simulink model "MaIA_SDCI_Temperature_Control"  (R2025b)
settings: Solver=VariableStepAuto  StartTime=0.0  StopTime=1800  RelTol=1e-3
PreLoadFcn:
  | %% MaIA_SDCI - Model Preload Callback
  | % Keep this callback intentionally minimal.
  | % All portable initialization logic lives in startup_project.m.
  | 
  | modelFile = get_param(bdroot, 'FileName');
  | 
  | if isempty(modelFile)
  |     error('MaIA_SDCI:ModelFileNotFound', ...
  |         'Unable to determine the current model file location.');
  | end
  | 
  | projectRoot = fileparts(modelFile);
  | addpath(projectRoot, '-begin');
  | rehash path;
  | startup_project(projectRoot);
InitFcn:
  | %% ============================================================
  | %  SIMULATION LAUNCH SOURCE
  | %  ============================================================
  | 
  | % false -> Run initiated directly from Simulink
  | % true  -> Run initiated from the MaIA_SDCI GUI
  | %
  | % Do not overwrite this variable if it already exists because
  | % the GUI sets it to true immediately before starting a run.
  | 
  | if ~evalin( ...
  |         'base', ...
  |         'exist(''MaIA_SDCI_RUN_FROM_GUI'',''var'')')
  | 
  |     assignin( ...
  |         'base', ...
  |         'MaIA_SDCI_RUN_FROM_GUI', ...
  |         false);
  | 
  | end
StartFcn:
  | %% MaIA_SDCI - Simulation Start Callback
  | 
  | runFromGUI = false;
  | 
  | %% Check simulation origin
  | 
  | if evalin( ...
  |         'base', ...
  |         'exist(''MaIA_SDCI_RUN_FROM_GUI'',''var'')')
  | 
  |     flagValue = evalin( ...
  |         'base', ...
  |         'MaIA_SDCI_RUN_FROM_GUI');
  | 
  |     if islogical(flagValue) || isnumeric(flagValue)
  |         runFromGUI = logical(flagValue);
  |     end
  | 
  | end
  | 
  | %% Open or focus the control application
  | 
  | launch_app;
  | 
  | %% Manual Run from Simulink
  | 
  | if ~runFromGUI
  | 
  |     drawnow;
  | 
  |     set_param( ...
  |         bdroot, ...
  |         'SimulationCommand', ...
  |         'stop');
  | 
  | end
values from neighbouring files (symbols this model uses):
  CFG = project_config()    [startup_project.m]
  ENV = environment_parameters()    [startup_project.m]
  MODEL = model_parameters()    [startup_project.m]
  SENSOR = sensor_parameters()    [startup_project.m]
libraries: fl_lib x58, nesl_utility x38, simulink x2
(part 1 of 2)
settings Model: PacingRate=100  Creator=leffe  LastModifiedBy=leffe

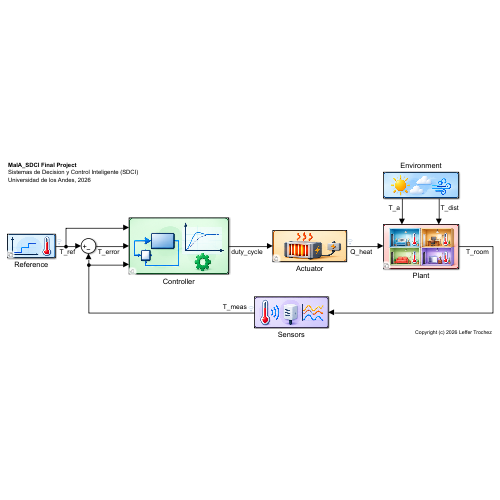
[thumbnail: Simulink's stored preview of the top-level diagram]
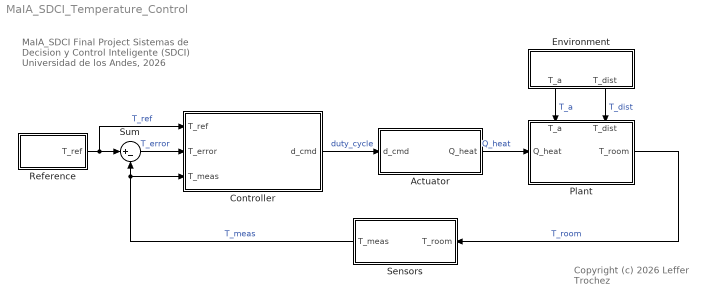
== system MaIA_SDCI_Temperature_Control ==
  note: Copyright (c) 2026 Leffer Trochez
  note: MaIA_SDCI Final Project
      | Sistemas de Decision y Control Inteligente (SDCI)
      | Universidad de los Andes, 2026
  Actuator : Subsystem  Variant=on  AllowFlexibleInterface=off
      mask Display: image('Actuador.png');
  Controller : Subsystem  Variant=on  AllowFlexibleInterface=off
      mask Display: image('Controller.png');
  Environment : Subsystem
      settings: PortSchema="{\"entries\":[{\"content\":{\"sides\":[{\"content\":{},\"type\":\"ConnectorPlacement.EquallySpacedRectSide\",\"uuid\":\"1a7bcca7-25d4-42c2-aca3-18b46478235c\"},{\"content\":{\"side\":\"RIGHT\"},\"type\":\"ConnectorPlacement.EquallySpacedRectSide\",\"uuid\":\"da09975b-28e2-4b16-92a5-057e0d52e938\"},{\"content\":{\"side\":\"TOP\"},\"type\":\"ConnectorPlacement.EquallySpacedRectSide\",\"uuid\":\"de133f6c-3388-4fad-acff-8d704dc07206\"},{\"content\":{\"connectorIds\":[\"Out1\",\"Out2\"],\"side\":\"BOTTOM\"},\"type\":\"ConnectorPlacement.EquallySpacedRectSide\",\"uuid\":\"319bfc7a-61e7-4d85-9757-ec8360a08b79\"}]},\"type\":\"ConnectorPlacement.EquallySpacedConnector\",\"uuid\":\"d277b6ce-17a2-42f7-b477-40e753a041d0\"}],\"packageUris\":[\"http://schema.mathworks.com/mf0/Connector/R2020b\"],\"version\":\"1.0\"}"
      mask Display: image('Environment.png');
  Plant : Subsystem  Variant=on  AllowFlexibleInterface=off
      settings: PortSchema="{\"entries\":[{\"content\":{\"sides\":[{\"content\":{\"connectorIds\":[\"In1\"]},\"type\":\"ConnectorPlacement.EquallySpacedRectSide\",\"uuid\":\"eba42224-8341-45a9-ac01-2acfcdf2210a\"},{\"content\":{\"connectorIds\":[\"Out1\"],\"side\":\"RIGHT\"},\"type\":\"ConnectorPlacement.EquallySpacedRectSide\",\"uuid\":\"282eb00b-7a70-45a6-85b7-dc180b696deb\"},{\"content\":{\"connectorIds\":[\"In2\",\"In3\"],\"side\":\"TOP\"},\"type\":\"ConnectorPlacement.EquallySpacedRectSide\",\"uuid\":\"41565600-1cc1-40b4-b112-8c0c6227dbf3\"}]},\"type\":\"ConnectorPlacement.EquallySpacedConnector\",\"uuid\":\"88025b6d-ed49-4509-ac82-02d3bec1907f\"}],\"packageUris\":[\"http://schema.mathworks.com/mf0/Connector/R2020b\"],\"version\":\"1.0\"}"
      mask Display: image('Plant.png');
  Reference : Subsystem  Variant=on  AllowFlexibleInterface=off
      mask Display: image('Reference.png');
  Sensors : Subsystem
      mask Display: image('Sensor.png');
  Sum : Sum  Inputs=|+-
  wires:
  Reference/1(T_ref) -> Sum/1, Controller/1(T_ref)  "T_ref"
  Sum/1 -> Controller/2(T_error)  "T_error"
  Sensors/1(T_meas) -> Controller/3(T_meas), Sum/2  "T_meas"
  Controller/1(d_cmd) -> Actuator/1(d_cmd)  "duty_cycle"
  Actuator/1(Q_heat) -> Plant/1(Q_heat)  "Q_heat"
  Plant/1(T_room) -> Sensors/1(T_room)  "T_room"
  Environment/1(T_a) -> Plant/2(T_a)  "T_a"
  Environment/2(T_dist) -> Plant/3(T_dist)  "T_dist"

== system MaIA_SDCI_Temperature_Control/Actuator ==
  d_cmd : Inport
  Block_Based : Subsystem  VariantControl=MODEL_TYPE_ID == 1
  Physics_Based : Subsystem  VariantControl=MODEL_TYPE_ID == 2
  Q_heat : Outport

== system MaIA_SDCI_Temperature_Control/Controller ==
  T_ref : Inport
  T_error : Inport  Port=2
  T_meas : Inport  Port=3
  Extremum_Seeking_Control : Subsystem  VariantControl=CONTROLLER_ID == 4
  Fuzzy_Logic : Subsystem  VariantControl=CONTROLLER_ID == 2
  Model_Predictive_Control : Subsystem  VariantControl=CONTROLLER_ID == 3
  ON_OFF : Subsystem  VariantControl=CONTROLLER_ID == 1
  Replicator_Dynamics : Subsystem  VariantControl=CONTROLLER_ID == 5
  d_cmd : Outport

== system MaIA_SDCI_Temperature_Control/Environment ==
  Ambient Temperature : Constant  Value=ENV.T_a
  Disturbance End : Step  Time=60 * ENV.disturbance.endTime  After=-ENV.disturbance.enabled * ENV.disturbance.amplitude  SampleTime=0
  Disturbance Start : Step  Time=60 * ENV.disturbance.startTime  After=ENV.disturbance.enabled * ENV.disturbance.amplitude  SampleTime=0
  Room Selection : Gain  Gain=ENV.disturbance.roomMask  Multiplication=Matrix(K*u)
  Temperature Disturbance : Sum  Inputs=|++
  T_a : Outport
  T_dist : Outport  Port=2
  tag scope: T_a=global
  wires:
  Ambient Temperature/1 -> [T_a], T_a/1
  Disturbance Start/1 -> Temperature Disturbance/1
  Disturbance End/1 -> Temperature Disturbance/2
  Temperature Disturbance/1 -> Room Selection/1
  Room Selection/1 -> T_dist/1

== system MaIA_SDCI_Temperature_Control/Plant ==
  Q_heat : Inport
  T_a : Inport  Port=2
  T_dist : Inport  Port=3
  Block_Based : Subsystem  VariantControl=MODEL_TYPE_ID == 1
  Physics_Based : Subsystem  VariantControl=MODEL_TYPE_ID == 2
  T_room : Outport

== system MaIA_SDCI_Temperature_Control/Reference ==
  Reference_1Room : Subsystem  VariantControl=CONTROLLER_ID == 4
  Reference_4Rooms : Subsystem  VariantControl=CONTROLLER_ID ~= 4
  T_ref : Outport

== system MaIA_SDCI_Temperature_Control/Sensors ==
  T_room : Inport
  Active Sensor Mask : Product
  Demux : Demux
  Mux : Mux
  Sensor Mask : Constant  Value=[1; CONTROLLER_ID ~= 4; CONTROLLER_ID ~= 4; CONTROLLER_ID ~= 4]
  Temperature Sensor 1 : Subsystem
  Temperature Sensor 2 : Subsystem
  Temperature Sensor 3 : Subsystem
  Temperature Sensor 4 : Subsystem
  T_meas : Outport
  wires:
  T_room/1 -> Demux/1
  Temperature Sensor 1/1(T_meas_1) -> Mux/1
  Demux/1 -> Temperature Sensor 1/1(T_1)
  Mux/1 -> Active Sensor Mask/1
  Sensor Mask/1 -> Active Sensor Mask/2
  Active Sensor Mask/1 -> T_meas/1
  Demux/2 -> Temperature Sensor 2/1(T_2)
  Demux/3 -> Temperature Sensor 3/1(T_3)
  Demux/4 -> Temperature Sensor 4/1(T_4)
  Temperature Sensor 2/1(T_meas_2) -> Mux/2
  Temperature Sensor 3/1(T_meas_3) -> Mux/3
  Temperature Sensor 4/1(T_meas_4) -> Mux/4

== system MaIA_SDCI_Temperature_Control/Actuator/Block_Based ==
  d_cmd : Inport
  Constant : Constant
  Constant1 : Constant  Value=0
  Demux : Demux
  Heater_1 : Subsystem
  Heater_2 : Subsystem
  Heater_3 : Subsystem
  Heater_4 : Subsystem
  Mux : Mux
  "Saturation Dynamic " : simulink/Discontinuities/Saturation Dynamic  OutMin=[]  OutMax=[]  OutDataTypeStr=Inherit: Same as second input  OutDataType=fixdt(1, 16)  OutScaling=2^-10  DoSatur=off
  Q_heat : Outport
  wires:
  Mux/1 -> Q_heat/1  "[W]"
  "Saturation Dynamic "/1 -> Demux/1  "[-]"
  d_cmd/1 -> "Saturation Dynamic "/2
  Demux/1 -> Heater_1/1(d_1)
  Heater_1/1(Q_1) -> Mux/1
  Constant/1 -> "Saturation Dynamic "/1
  Constant1/1 -> "Saturation Dynamic "/3
  Demux/2 -> Heater_2/1(d_2)
  Demux/3 -> Heater_3/1(d_3)
  Demux/4 -> Heater_4/1(d_4)
  Heater_2/1(Q_2) -> Mux/2
  Heater_3/1(Q_3) -> Mux/3
  Heater_4/1(Q_4) -> Mux/4

== system MaIA_SDCI_Temperature_Control/Actuator/Physics_Based ==
  d_cmd : Inport
  Demux : Demux
  "Duty Cycle Saturation " : simulink/Discontinuities/Saturation Dynamic  OutMin=[]  OutMax=[]  OutDataTypeStr=Inherit: Same as second input  OutDataType=fixdt(1, 16)  OutScaling=2^-10  DoSatur=off
  Heater_1 : Subsystem
  Heater_2 : Subsystem
  Heater_3 : Subsystem
  Heater_4 : Subsystem
  Lower Duty Limit : Constant  Value=0
  Mux : Mux
  Upper Duty Limit : Constant
  Q_heat : Outport
  wires:
  d_cmd/1 -> "Duty Cycle Saturation "/2
  Lower Duty Limit/1 -> "Duty Cycle Saturation "/3
  Heater_1/1(Q_1) -> Mux/1
  Upper Duty Limit/1 -> "Duty Cycle Saturation "/1
  Mux/1 -> Q_heat/1  "[W]"
  Demux/1 -> Heater_1/1(d_1)
  "Duty Cycle Saturation "/1 -> Demux/1  "[-]"
  Demux/2 -> Heater_2/1(d_2)
  Demux/3 -> Heater_3/1(d_3)
  Demux/4 -> Heater_4/1(d_4)
  Heater_2/1(Q_2) -> Mux/2
  Heater_3/1(Q_3) -> Mux/3
  Heater_4/1(Q_4) -> Mux/4

== system MaIA_SDCI_Temperature_Control/Controller/Extremum_Seeking_Control ==
  T_ref : Inport
  T_error : Inport  Port=2
  T_meas : Inport  Port=3
  d_cmd : Outport

== system MaIA_SDCI_Temperature_Control/Controller/Fuzzy_Logic ==
  T_ref : Inport
  T_error : Inport  Port=2
  T_meas : Inport  Port=3
  d_cmd : Outport

== system MaIA_SDCI_Temperature_Control/Controller/Model_Predictive_Control ==
  T_ref : Inport
  T_error : Inport  Port=2
  T_meas : Inport  Port=3
  d_cmd : Outport

== system MaIA_SDCI_Temperature_Control/Controller/ON_OFF ==
  T_ref : Inport
  T_error : Inport  Port=2
  T_meas : Inport  Port=3
  d_cmd : Outport

== system MaIA_SDCI_Temperature_Control/Controller/Replicator_Dynamics ==
  T_ref : Inport
  T_error : Inport  Port=2
  T_meas : Inport  Port=3
  d_cmd : Outport

== system MaIA_SDCI_Temperature_Control/Plant/Block_Based ==
  Q_heat : Inport
  T_a : Inport  Port=2
  T_dist : Inport  Port=3
  Building Configuration : Subsystem  Variant=on  AllowFlexibleInterface=off
  T_room : Outport
  wires:
  Building Configuration/1(T_room) -> T_room/1
  Q_heat/1 -> Building Configuration/1(Q_heat)
  T_a/1 -> Building Configuration/2(T_a)
  T_dist/1 -> Building Configuration/3(T_dist)

== system MaIA_SDCI_Temperature_Control/Plant/Physics_Based ==
  Q_heat : Inport
  T_a : Inport  Port=2
  T_dist : Inport  Port=3
  Building Configuration : Subsystem  Variant=on  AllowFlexibleInterface=off
  T_room : Outport
  wires:
  Q_heat/1 -> Building Configuration/1(Q_heat)
  T_a/1 -> Building Configuration/2(T_a)
  T_dist/1 -> Building Configuration/3(T_dist)
  Building Configuration/1(T_room) -> T_room/1

== system MaIA_SDCI_Temperature_Control/Reference/Reference_1Room ==
  Constant : Constant  Value=[CFG.reference.singleRoom; 0; 0; 0]
  T_ref : Outport
  wires:
  Constant/1 -> T_ref/1

== system MaIA_SDCI_Temperature_Control/Reference/Reference_4Rooms ==
  Constant : Constant  Value=CFG.reference.fourRooms
  T_ref : Outport
  wires:
  Constant/1 -> T_ref/1

== system MaIA_SDCI_Temperature_Control/Sensors/Temperature Sensor 1 ==
  T_1 : Inport
  Measured Temperature : Sum  Inputs=|+++
  Measurement Noise : RandomNumber  Variance=SENSOR.noiseStd(1)^2  Seed=SENSOR.seed(1)  SampleTime=SENSOR.sampleTime
  Sampling : ZeroOrderHold  SampleTime=SENSOR.sampleTime
  Sensor Dynamics Gain : Gain  Gain=1/SENSOR.tau
  Sensor Temperature : Integrator  InitialCondition=SENSOR.initialTemperature(1)
  Sensor Bias : Constant  Value=SENSOR.bias(1)
  Sum : Sum  Inputs=|+-
  T_meas_1 : Outport
  wires:
  T_1/1 -> Sum/1
  Sensor Temperature/1 -> Sum/2, Sampling/1
  Sampling/1 -> Measured Temperature/2
  Sensor Bias/1 -> Measured Temperature/3
  Measurement Noise/1 -> Measured Temperature/1
  Measured Temperature/1 -> T_meas_1/1
  Sum/1 -> Sensor Dynamics Gain/1
  Sensor Dynamics Gain/1 -> Sensor Temperature/1

== system MaIA_SDCI_Temperature_Control/Sensors/Temperature Sensor 2 ==
  T_2 : Inport
  Measured Temperature : Sum  Inputs=|+++
  Measurement Noise : RandomNumber  Variance=SENSOR.noiseStd(2)^2  Seed=SENSOR.seed(2)  SampleTime=SENSOR.sampleTime
  Sampling : ZeroOrderHold  SampleTime=SENSOR.sampleTime
  Sensor Dynamics Gain : Gain  Gain=1/SENSOR.tau
  Sensor Temperature : Integrator  InitialCondition=SENSOR.initialTemperature(2)
  Sensor Bias : Constant  Value=SENSOR.bias(2)
  Sum : Sum  Inputs=|+-
  T_meas_2 : Outport
  wires:
  T_2/1 -> Sum/1
  Sum/1 -> Sensor Dynamics Gain/1
  Measured Temperature/1 -> T_meas_2/1
  Measurement Noise/1 -> Measured Temperature/1
  Sampling/1 -> Measured Temperature/2
  Sensor Temperature/1 -> Sum/2, Sampling/1
  Sensor Bias/1 -> Measured Temperature/3
  Sensor Dynamics Gain/1 -> Sensor Temperature/1

== system MaIA_SDCI_Temperature_Control/Sensors/Temperature Sensor 3 ==
  T_3 : Inport
  Measured Temperature : Sum  Inputs=|+++
  Measurement Noise : RandomNumber  Variance=SENSOR.noiseStd(3)^2  Seed=SENSOR.seed(3)  SampleTime=SENSOR.sampleTime
  Sampling : ZeroOrderHold  SampleTime=SENSOR.sampleTime
  Sensor Dynamics Gain : Gain  Gain=1/SENSOR.tau
  Sensor Temperature : Integrator  InitialCondition=SENSOR.initialTemperature(3)
  Sensor Bias : Constant  Value=SENSOR.bias(3)
  Sum : Sum  Inputs=|+-
  T_meas_3 : Outport
  wires:
  Sensor Dynamics Gain/1 -> Sensor Temperature/1
  Sampling/1 -> Measured Temperature/2
  Measured Temperature/1 -> T_meas_3/1
  Sum/1 -> Sensor Dynamics Gain/1
  T_3/1 -> Sum/1
  Sensor Bias/1 -> Measured Temperature/3
  Sensor Temperature/1 -> Sum/2, Sampling/1
  Measurement Noise/1 -> Measured Temperature/1

== system MaIA_SDCI_Temperature_Control/Sensors/Temperature Sensor 4 ==
  T_4 : Inport
  Measured Temperature : Sum  Inputs=|+++
  Measurement Noise : RandomNumber  Variance=SENSOR.noiseStd(4)^2  Seed=SENSOR.seed(4)  SampleTime=SENSOR.sampleTime
  Sampling : ZeroOrderHold  SampleTime=SENSOR.sampleTime
  Sensor Dynamics Gain : Gain  Gain=1/SENSOR.tau
  Sensor Temperature : Integrator  InitialCondition=SENSOR.initialTemperature(4)
  Sensor Bias : Constant  Value=SENSOR.bias(4)
  Sum : Sum  Inputs=|+-
  T_meas_4 : Outport
  wires:
  Sensor Temperature/1 -> Sum/2, Sampling/1
  Measurement Noise/1 -> Measured Temperature/1
  Sensor Bias/1 -> Measured Temperature/3
  T_4/1 -> Sum/1
  Sensor Dynamics Gain/1 -> Sensor Temperature/1
  Sum/1 -> Sensor Dynamics Gain/1
  Measured Temperature/1 -> T_meas_4/1
  Sampling/1 -> Measured Temperature/2

== system MaIA_SDCI_Temperature_Control/Actuator/Block_Based/Heater_1 ==
  d_1 : Inport
  Control Window Hold : ZeroOrderHold  SampleTime=MODEL.BLOCK_BASED.ACTUATOR.controlWindow
  Cycle Quantizer : Rounding  Operator=round
  Cycle Count to Thermal Power : Gain  Gain=|
      | MODEL.BLOCK_BASED.ACTUATOR.P_rated * MODEL.BLOCK_BASED.ACTUATOR.efficiency / ...
      |     MODEL.BLOCK_BASED.ACTUATOR.cyclesPerWindow
  Duty to Cycle Count : Gain  Gain=MODEL.BLOCK_BASED.ACTUATOR.cyclesPerWindow
  Q_1 : Outport
  wires:
  d_1/1 -> Control Window Hold/1
  Duty to Cycle Count/1 -> Cycle Quantizer/1
  Control Window Hold/1 -> Duty to Cycle Count/1
  Cycle Quantizer/1 -> Cycle Count to Thermal Power/1
  Cycle Count to Thermal Power/1 -> Q_1/1

== system MaIA_SDCI_Temperature_Control/Actuator/Block_Based/Heater_2 ==
  d_2 : Inport
  Control Window Hold : ZeroOrderHold  SampleTime=MODEL.BLOCK_BASED.ACTUATOR.controlWindow
  Cycle Quantizer : Rounding  Operator=round
  Cycle Count to Thermal Power : Gain  Gain=|
      | MODEL.BLOCK_BASED.ACTUATOR.P_rated * MODEL.BLOCK_BASED.ACTUATOR.efficiency / ...
      |     MODEL.BLOCK_BASED.ACTUATOR.cyclesPerWindow
  Duty to Cycle Count : Gain  Gain=MODEL.BLOCK_BASED.ACTUATOR.cyclesPerWindow
  Q_2 : Outport
  wires:
  Cycle Quantizer/1 -> Cycle Count to Thermal Power/1
  Control Window Hold/1 -> Duty to Cycle Count/1
  Duty to Cycle Count/1 -> Cycle Quantizer/1
  d_2/1 -> Control Window Hold/1
  Cycle Count to Thermal Power/1 -> Q_2/1

== system MaIA_SDCI_Temperature_Control/Actuator/Block_Based/Heater_3 ==
  d_3 : Inport
  Control Window Hold : ZeroOrderHold  SampleTime=MODEL.BLOCK_BASED.ACTUATOR.controlWindow
  Cycle Quantizer : Rounding  Operator=round
  Cycle Count to Thermal Power : Gain  Gain=|
      | MODEL.BLOCK_BASED.ACTUATOR.P_rated * MODEL.BLOCK_BASED.ACTUATOR.efficiency / ...
      |     MODEL.BLOCK_BASED.ACTUATOR.cyclesPerWindow
  Duty to Cycle Count : Gain  Gain=MODEL.BLOCK_BASED.ACTUATOR.cyclesPerWindow
  Q_3 : Outport
  wires:
  Cycle Quantizer/1 -> Cycle Count to Thermal Power/1
  Control Window Hold/1 -> Duty to Cycle Count/1
  Duty to Cycle Count/1 -> Cycle Quantizer/1
  d_3/1 -> Control Window Hold/1
  Cycle Count to Thermal Power/1 -> Q_3/1

== system MaIA_SDCI_Temperature_Control/Actuator/Block_Based/Heater_4 ==
  d_4 : Inport
  Control Window Hold : ZeroOrderHold  SampleTime=MODEL.BLOCK_BASED.ACTUATOR.controlWindow
  Cycle Quantizer : Rounding  Operator=round
  Cycle Count to Thermal Power : Gain  Gain=|
      | MODEL.BLOCK_BASED.ACTUATOR.P_rated * MODEL.BLOCK_BASED.ACTUATOR.efficiency / ...
      |     MODEL.BLOCK_BASED.ACTUATOR.cyclesPerWindow
  Duty to Cycle Count : Gain  Gain=MODEL.BLOCK_BASED.ACTUATOR.cyclesPerWindow
  Q_4 : Outport
  wires:
  Cycle Quantizer/1 -> Cycle Count to Thermal Power/1
  Control Window Hold/1 -> Duty to Cycle Count/1
  Duty to Cycle Count/1 -> Cycle Quantizer/1
  d_4/1 -> Control Window Hold/1
  Cycle Count to Thermal Power/1 -> Q_4/1

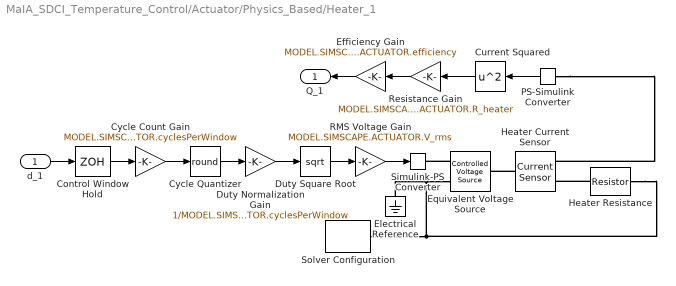
== system MaIA_SDCI_Temperature_Control/Actuator/Physics_Based/Heater_1 ==
  d_1 : Inport
  Control Window Hold : ZeroOrderHold  SampleTime=MODEL.SIMSCAPE.ACTUATOR.controlWindow
  Current Squared : Math  Operator=square
  Cycle Count Gain : Gain  Gain=MODEL.SIMSCAPE.ACTUATOR.cyclesPerWindow
  Cycle Quantizer : Rounding  Operator=round
  Duty Normalization Gain : Gain  Gain=1/MODEL.SIMSCAPE.ACTUATOR.cyclesPerWindow
  Duty Square Root : Sqrt
  Efficiency Gain : Gain  Gain=MODEL.SIMSCAPE.ACTUATOR.efficiency
  Electrical Reference : fl_lib/Electrical/Electrical Elements/Electrical Reference
  Equivalent Voltage Source : fl_lib/Electrical/Electrical Sources/Controlled Voltage Source
  Heater Resistance : fl_lib/Electrical/Electrical Elements/Resistor  R=MODEL.SIMSCAPE.ACTUATOR.R_heater Ohm  i_specify=off  i_priority=None  i=0 A  i_nominal_specify=off  i_nominal_value=1  i_nominal_unit=A  v_specify=off  v_priority=None  v=0 V  v_nominal_specify=off  v_nominal_value=1  v_nominal_unit=V
  Heater Current Sensor : fl_lib/Electrical/Electrical Sensors/Current Sensor
  PS-Simulink Converter : nesl_utility/PS-Simulink Converter  PhysicalDomain=network_engine_domain  SubClassName=ps_output  LeftPortType=input  RightPortType=output  PseudoPeriodic=off  Frequencies=[]  VectorFormat=inherit  Unit=A  AffineConversion=off
  RMS Voltage Gain : Gain  Gain=MODEL.SIMSCAPE.ACTUATOR.V_rms
  Resistance Gain : Gain  Gain=MODEL.SIMSCAPE.ACTUATOR.R_heater
  Simulink-PS Converter : nesl_utility/Simulink-PS Converter  PhysicalDomain=network_engine_domain  SubClassName=ps_input  LeftPortType=input  RightPortType=output  PseudoPeriodic=off  Frequencies=[]  NoiseDistribution=none  NoiseParameters=[]  Unit=V  AffineConversion=off  FilteringAndDerivatives=provide  SimscapeFilterOrder=1  InputFilterTimeConstant=0.001  UdotUserProvided=0
  Solver Configuration : nesl_utility/Solver Configuration  PhysicalDomain=network_engine_domain  SubClassName=solver  LeftPortType=input  RightPortType=generic  Tones=[]  Harmonics=[]  SimulateNoise=off  Profile=off  UseLocalSampling=off  EnableSwitchedLinearOptims=on  FrequencyDomain=off  UseCCode=off  RelTol=0.001  AbsTol=0.001  MinStep=1e-09  ToWorkspace=off  RevertToSquareIcSolve=off  NumHomotopyIterations=100  PhasorMode=off  PhasorModeNumHarmonics=1  ConsistencySolver=NEWTON_XTOL_AFTER_FTOL  IndexReductionMethod=DerivativeReplacement  DoDC=off  ResidualTolerance=1e-09  ConsistencyTolSource=GLOBAL  ConsistencyAbsTol=0.001  ConsistencyRelTol=0.001  ConsistencyTolFactor=0.001  UseLocalSolver=off  LocalSolverChoice=NE_BACKWARD_EULER_ADVANCER  ResolveIndetEquations=on  FunctionEvalNumThread=1  LocalSolverSampleTime=0.001  DoFixedCost=off  MaxNonlinIter=3  MaxModeIter=2  ComputeImpulses=off  ImpulseIterations=2  LinearAlgebra=auto  LinearAlgebraNumThread=0  EquationFormulation=NE_TIME_EF  DelaysMemoryBudget=1024  AutomaticFiltering=on  FilteringTimeConstant=0.001  PartitionStorageMethod=AS_NEEDED  PartitionMemoryBudget=1024  PartitionMethod=ROBUST  MultibodyUseLocalSolver=off  MultibodyLocalSolverChoice=ODE1  MultibodyLocalSolverSampleTime=0.001
  Q_1 : Outport
  wires:
  d_1/1 -> Control Window Hold/1
  Cycle Count Gain/1 -> Cycle Quantizer/1
  Control Window Hold/1 -> Cycle Count Gain/1
  Cycle Quantizer/1 -> Duty Normalization Gain/1
  Duty Normalization Gain/1 -> Duty Square Root/1
  Duty Square Root/1 -> RMS Voltage Gain/1
  RMS Voltage Gain/1 -> Simulink-PS Converter/1
  PS-Simulink Converter/1 -> Current Squared/1
  Current Squared/1 -> Resistance Gain/1
  Resistance Gain/1 -> Efficiency Gain/1
  Efficiency Gain/1 -> Q_1/1
  connections:
  Equivalent Voltage Source/RConn1 -- Simulink-PS Converter/RConn1
  Heater Current Sensor/LConn1 -- Equivalent Voltage Source/LConn1
  Heater Resistance/LConn1 -- Heater Current Sensor/RConn2
  Heater Resistance/RConn1 -- Electrical Reference/LConn1 -- Equivalent Voltage Source/RConn2 -- Solver Configuration/RConn1
  PS-Simulink Converter/LConn1 -- Heater Current Sensor/RConn1

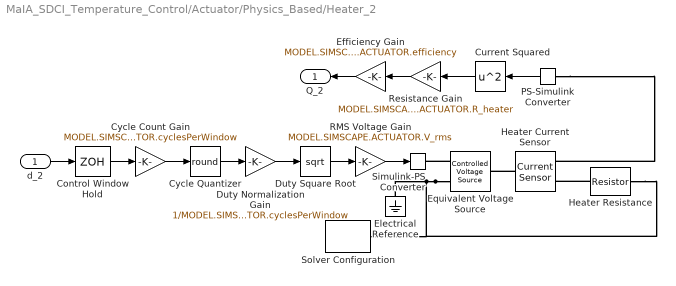
== system MaIA_SDCI_Temperature_Control/Actuator/Physics_Based/Heater_2 ==
  d_2 : Inport
  Control Window Hold : ZeroOrderHold  SampleTime=MODEL.SIMSCAPE.ACTUATOR.controlWindow
  Current Squared : Math  Operator=square
  Cycle Count Gain : Gain  Gain=MODEL.SIMSCAPE.ACTUATOR.cyclesPerWindow
  Cycle Quantizer : Rounding  Operator=round
  Duty Normalization Gain : Gain  Gain=1/MODEL.SIMSCAPE.ACTUATOR.cyclesPerWindow
  Duty Square Root : Sqrt
  Efficiency Gain : Gain  Gain=MODEL.SIMSCAPE.ACTUATOR.efficiency
  Electrical Reference : fl_lib/Electrical/Electrical Elements/Electrical Reference
  Equivalent Voltage Source : fl_lib/Electrical/Electrical Sources/Controlled Voltage Source
  Heater Resistance : fl_lib/Electrical/Electrical Elements/Resistor  R=MODEL.SIMSCAPE.ACTUATOR.R_heater Ohm  i_specify=off  i_priority=None  i=0 A  i_nominal_specify=off  i_nominal_value=1  i_nominal_unit=A  v_specify=off  v_priority=None  v=0 V  v_nominal_specify=off  v_nominal_value=1  v_nominal_unit=V
  Heater Current Sensor : fl_lib/Electrical/Electrical Sensors/Current Sensor
  PS-Simulink Converter : nesl_utility/PS-Simulink Converter  PhysicalDomain=network_engine_domain  SubClassName=ps_output  LeftPortType=input  RightPortType=output  PseudoPeriodic=off  Frequencies=[]  VectorFormat=inherit  Unit=A  AffineConversion=off
  RMS Voltage Gain : Gain  Gain=MODEL.SIMSCAPE.ACTUATOR.V_rms
  Resistance Gain : Gain  Gain=MODEL.SIMSCAPE.ACTUATOR.R_heater
  Simulink-PS Converter : nesl_utility/Simulink-PS Converter  PhysicalDomain=network_engine_domain  SubClassName=ps_input  LeftPortType=input  RightPortType=output  PseudoPeriodic=off  Frequencies=[]  NoiseDistribution=none  NoiseParameters=[]  Unit=V  AffineConversion=off  FilteringAndDerivatives=provide  SimscapeFilterOrder=1  InputFilterTimeConstant=0.001  UdotUserProvided=0
  Solver Configuration : nesl_utility/Solver Configuration  PhysicalDomain=network_engine_domain  SubClassName=solver  LeftPortType=input  RightPortType=generic  Tones=[]  Harmonics=[]  SimulateNoise=off  Profile=off  UseLocalSampling=off  EnableSwitchedLinearOptims=on  FrequencyDomain=off  UseCCode=off  RelTol=0.001  AbsTol=0.001  MinStep=1e-09  ToWorkspace=off  RevertToSquareIcSolve=off  NumHomotopyIterations=100  PhasorMode=off  PhasorModeNumHarmonics=1  ConsistencySolver=NEWTON_XTOL_AFTER_FTOL  IndexReductionMethod=DerivativeReplacement  DoDC=off  ResidualTolerance=1e-09  ConsistencyTolSource=GLOBAL  ConsistencyAbsTol=0.001  ConsistencyRelTol=0.001  ConsistencyTolFactor=0.001  UseLocalSolver=off  LocalSolverChoice=NE_BACKWARD_EULER_ADVANCER  ResolveIndetEquations=on  FunctionEvalNumThread=1  LocalSolverSampleTime=0.001  DoFixedCost=off  MaxNonlinIter=3  MaxModeIter=2  ComputeImpulses=off  ImpulseIterations=2  LinearAlgebra=auto  LinearAlgebraNumThread=0  EquationFormulation=NE_TIME_EF  DelaysMemoryBudget=1024  AutomaticFiltering=on  FilteringTimeConstant=0.001  PartitionStorageMethod=AS_NEEDED  PartitionMemoryBudget=1024  PartitionMethod=ROBUST  MultibodyUseLocalSolver=off  MultibodyLocalSolverChoice=ODE1  MultibodyLocalSolverSampleTime=0.001
  Q_2 : Outport
  wires:
  d_2/1 -> Control Window Hold/1
  Duty Normalization Gain/1 -> Duty Square Root/1
  Resistance Gain/1 -> Efficiency Gain/1
  Current Squared/1 -> Resistance Gain/1
  PS-Simulink Converter/1 -> Current Squared/1
  RMS Voltage Gain/1 -> Simulink-PS Converter/1
  Cycle Quantizer/1 -> Duty Normalization Gain/1
  Duty Square Root/1 -> RMS Voltage Gain/1
  Efficiency Gain/1 -> Q_2/1
  Control Window Hold/1 -> Cycle Count Gain/1
  Cycle Count Gain/1 -> Cycle Quantizer/1
  connections:
  Equivalent Voltage Source/RConn2 -- Heater Resistance/RConn1 -- Solver Configuration/RConn1 -- Electrical Reference/LConn1
  Heater Current Sensor/LConn1 -- Equivalent Voltage Source/LConn1
  Equivalent Voltage Source/RConn1 -- Simulink-PS Converter/RConn1
  PS-Simulink Converter/LConn1 -- Heater Current Sensor/RConn1
  Heater Resistance/LConn1 -- Heater Current Sensor/RConn2

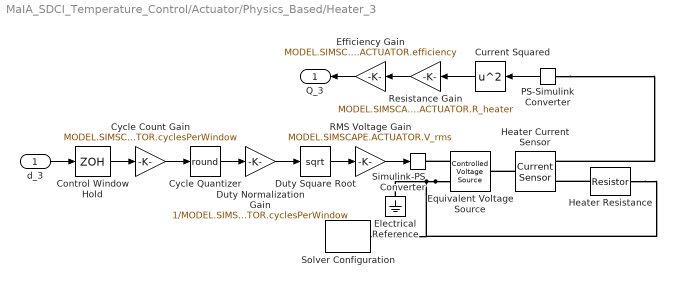
== system MaIA_SDCI_Temperature_Control/Actuator/Physics_Based/Heater_3 ==
  d_3 : Inport
  Control Window Hold : ZeroOrderHold  SampleTime=MODEL.SIMSCAPE.ACTUATOR.controlWindow
  Current Squared : Math  Operator=square
  Cycle Count Gain : Gain  Gain=MODEL.SIMSCAPE.ACTUATOR.cyclesPerWindow
  Cycle Quantizer : Rounding  Operator=round
  Duty Normalization Gain : Gain  Gain=1/MODEL.SIMSCAPE.ACTUATOR.cyclesPerWindow
  Duty Square Root : Sqrt
  Efficiency Gain : Gain  Gain=MODEL.SIMSCAPE.ACTUATOR.efficiency
  Electrical Reference : fl_lib/Electrical/Electrical Elements/Electrical Reference
  Equivalent Voltage Source : fl_lib/Electrical/Electrical Sources/Controlled Voltage Source
  Heater Resistance : fl_lib/Electrical/Electrical Elements/Resistor  R=MODEL.SIMSCAPE.ACTUATOR.R_heater Ohm  i_specify=off  i_priority=None  i=0 A  i_nominal_specify=off  i_nominal_value=1  i_nominal_unit=A  v_specify=off  v_priority=None  v=0 V  v_nominal_specify=off  v_nominal_value=1  v_nominal_unit=V
  Heater Current Sensor : fl_lib/Electrical/Electrical Sensors/Current Sensor
  PS-Simulink Converter : nesl_utility/PS-Simulink Converter  PhysicalDomain=network_engine_domain  SubClassName=ps_output  LeftPortType=input  RightPortType=output  PseudoPeriodic=off  Frequencies=[]  VectorFormat=inherit  Unit=A  AffineConversion=off
  RMS Voltage Gain : Gain  Gain=MODEL.SIMSCAPE.ACTUATOR.V_rms
  Resistance Gain : Gain  Gain=MODEL.SIMSCAPE.ACTUATOR.R_heater
  Simulink-PS Converter : nesl_utility/Simulink-PS Converter  PhysicalDomain=network_engine_domain  SubClassName=ps_input  LeftPortType=input  RightPortType=output  PseudoPeriodic=off  Frequencies=[]  NoiseDistribution=none  NoiseParameters=[]  Unit=V  AffineConversion=off  FilteringAndDerivatives=provide  SimscapeFilterOrder=1  InputFilterTimeConstant=0.001  UdotUserProvided=0
  Solver Configuration : nesl_utility/Solver Configuration  PhysicalDomain=network_engine_domain  SubClassName=solver  LeftPortType=input  RightPortType=generic  Tones=[]  Harmonics=[]  SimulateNoise=off  Profile=off  UseLocalSampling=off  EnableSwitchedLinearOptims=on  FrequencyDomain=off  UseCCode=off  RelTol=0.001  AbsTol=0.001  MinStep=1e-09  ToWorkspace=off  RevertToSquareIcSolve=off  NumHomotopyIterations=100  PhasorMode=off  PhasorModeNumHarmonics=1  ConsistencySolver=NEWTON_XTOL_AFTER_FTOL  IndexReductionMethod=DerivativeReplacement  DoDC=off  ResidualTolerance=1e-09  ConsistencyTolSource=GLOBAL  ConsistencyAbsTol=0.001  ConsistencyRelTol=0.001  ConsistencyTolFactor=0.001  UseLocalSolver=off  LocalSolverChoice=NE_BACKWARD_EULER_ADVANCER  ResolveIndetEquations=on  FunctionEvalNumThread=1  LocalSolverSampleTime=0.001  DoFixedCost=off  MaxNonlinIter=3  MaxModeIter=2  ComputeImpulses=off  ImpulseIterations=2  LinearAlgebra=auto  LinearAlgebraNumThread=0  EquationFormulation=NE_TIME_EF  DelaysMemoryBudget=1024  AutomaticFiltering=on  FilteringTimeConstant=0.001  PartitionStorageMethod=AS_NEEDED  PartitionMemoryBudget=1024  PartitionMethod=ROBUST  MultibodyUseLocalSolver=off  MultibodyLocalSolverChoice=ODE1  MultibodyLocalSolverSampleTime=0.001
  Q_3 : Outport
  wires:
  d_3/1 -> Control Window Hold/1
  Duty Normalization Gain/1 -> Duty Square Root/1
  Resistance Gain/1 -> Efficiency Gain/1
  Current Squared/1 -> Resistance Gain/1
  PS-Simulink Converter/1 -> Current Squared/1
  RMS Voltage Gain/1 -> Simulink-PS Converter/1
  Cycle Quantizer/1 -> Duty Normalization Gain/1
  Duty Square Root/1 -> RMS Voltage Gain/1
  Efficiency Gain/1 -> Q_3/1
  Control Window Hold/1 -> Cycle Count Gain/1
  Cycle Count Gain/1 -> Cycle Quantizer/1
  connections:
  Equivalent Voltage Source/RConn2 -- Heater Resistance/RConn1 -- Solver Configuration/RConn1 -- Electrical Reference/LConn1
  Heater Current Sensor/LConn1 -- Equivalent Voltage Source/LConn1
  Equivalent Voltage Source/RConn1 -- Simulink-PS Converter/RConn1
  PS-Simulink Converter/LConn1 -- Heater Current Sensor/RConn1
  Heater Resistance/LConn1 -- Heater Current Sensor/RConn2

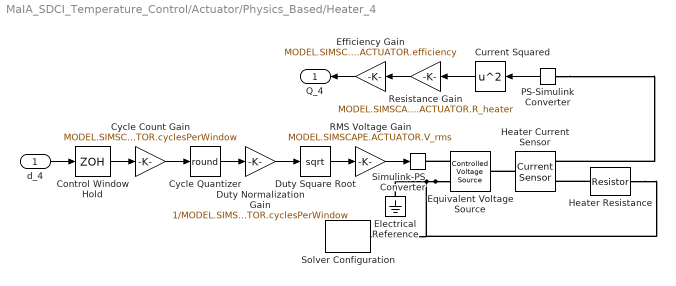
== system MaIA_SDCI_Temperature_Control/Actuator/Physics_Based/Heater_4 ==
  d_4 : Inport
  Control Window Hold : ZeroOrderHold  SampleTime=MODEL.SIMSCAPE.ACTUATOR.controlWindow
  Current Squared : Math  Operator=square
  Cycle Count Gain : Gain  Gain=MODEL.SIMSCAPE.ACTUATOR.cyclesPerWindow
  Cycle Quantizer : Rounding  Operator=round
  Duty Normalization Gain : Gain  Gain=1/MODEL.SIMSCAPE.ACTUATOR.cyclesPerWindow
  Duty Square Root : Sqrt
  Efficiency Gain : Gain  Gain=MODEL.SIMSCAPE.ACTUATOR.efficiency
  Electrical Reference : fl_lib/Electrical/Electrical Elements/Electrical Reference
  Equivalent Voltage Source : fl_lib/Electrical/Electrical Sources/Controlled Voltage Source
  Heater Resistance : fl_lib/Electrical/Electrical Elements/Resistor  R=MODEL.SIMSCAPE.ACTUATOR.R_heater Ohm  i_specify=off  i_priority=None  i=0 A  i_nominal_specify=off  i_nominal_value=1  i_nominal_unit=A  v_specify=off  v_priority=None  v=0 V  v_nominal_specify=off  v_nominal_value=1  v_nominal_unit=V
  Heater Current Sensor : fl_lib/Electrical/Electrical Sensors/Current Sensor
  PS-Simulink Converter : nesl_utility/PS-Simulink Converter  PhysicalDomain=network_engine_domain  SubClassName=ps_output  LeftPortType=input  RightPortType=output  PseudoPeriodic=off  Frequencies=[]  VectorFormat=inherit  Unit=A  AffineConversion=off
  RMS Voltage Gain : Gain  Gain=MODEL.SIMSCAPE.ACTUATOR.V_rms
  Resistance Gain : Gain  Gain=MODEL.SIMSCAPE.ACTUATOR.R_heater
  Simulink-PS Converter : nesl_utility/Simulink-PS Converter  PhysicalDomain=network_engine_domain  SubClassName=ps_input  LeftPortType=input  RightPortType=output  PseudoPeriodic=off  Frequencies=[]  NoiseDistribution=none  NoiseParameters=[]  Unit=V  AffineConversion=off  FilteringAndDerivatives=provide  SimscapeFilterOrder=1  InputFilterTimeConstant=0.001  UdotUserProvided=0
  Solver Configuration : nesl_utility/Solver Configuration  PhysicalDomain=network_engine_domain  SubClassName=solver  LeftPortType=input  RightPortType=generic  Tones=[]  Harmonics=[]  SimulateNoise=off  Profile=off  UseLocalSampling=off  EnableSwitchedLinearOptims=on  FrequencyDomain=off  UseCCode=off  RelTol=0.001  AbsTol=0.001  MinStep=1e-09  ToWorkspace=off  RevertToSquareIcSolve=off  NumHomotopyIterations=100  PhasorMode=off  PhasorModeNumHarmonics=1  ConsistencySolver=NEWTON_XTOL_AFTER_FTOL  IndexReductionMethod=DerivativeReplacement  DoDC=off  ResidualTolerance=1e-09  ConsistencyTolSource=GLOBAL  ConsistencyAbsTol=0.001  ConsistencyRelTol=0.001  ConsistencyTolFactor=0.001  UseLocalSolver=off  LocalSolverChoice=NE_BACKWARD_EULER_ADVANCER  ResolveIndetEquations=on  FunctionEvalNumThread=1  LocalSolverSampleTime=0.001  DoFixedCost=off  MaxNonlinIter=3  MaxModeIter=2  ComputeImpulses=off  ImpulseIterations=2  LinearAlgebra=auto  LinearAlgebraNumThread=0  EquationFormulation=NE_TIME_EF  DelaysMemoryBudget=1024  AutomaticFiltering=on  FilteringTimeConstant=0.001  PartitionStorageMethod=AS_NEEDED  PartitionMemoryBudget=1024  PartitionMethod=ROBUST  MultibodyUseLocalSolver=off  MultibodyLocalSolverChoice=ODE1  MultibodyLocalSolverSampleTime=0.001
  Q_4 : Outport
  wires:
  d_4/1 -> Control Window Hold/1
  Duty Normalization Gain/1 -> Duty Square Root/1
  Resistance Gain/1 -> Efficiency Gain/1
  Current Squared/1 -> Resistance Gain/1
  PS-Simulink Converter/1 -> Current Squared/1
  RMS Voltage Gain/1 -> Simulink-PS Converter/1
  Cycle Quantizer/1 -> Duty Normalization Gain/1
  Duty Square Root/1 -> RMS Voltage Gain/1
  Efficiency Gain/1 -> Q_4/1
  Control Window Hold/1 -> Cycle Count Gain/1
  Cycle Count Gain/1 -> Cycle Quantizer/1
  connections:
  Equivalent Voltage Source/RConn2 -- Heater Resistance/RConn1 -- Solver Configuration/RConn1 -- Electrical Reference/LConn1
  Heater Current Sensor/LConn1 -- Equivalent Voltage Source/LConn1
  Equivalent Voltage Source/RConn1 -- Simulink-PS Converter/RConn1
  PS-Simulink Converter/LConn1 -- Heater Current Sensor/RConn1
  Heater Resistance/LConn1 -- Heater Current Sensor/RConn2

== system MaIA_SDCI_Temperature_Control/Plant/Block_Based/Building Configuration ==
  Q_heat : Inport
  T_a : Inport  Port=2
  T_dist : Inport  Port=3
  Four_Rooms : Subsystem  VariantControl=CONTROLLER_ID ~= 4
  Single_Room : Subsystem  VariantControl=CONTROLLER_ID == 4
  T_room : Outport

== system MaIA_SDCI_Temperature_Control/Plant/Physics_Based/Building Configuration ==
  Q_heat : Inport
  T_a : Inport  Port=2
  T_dist : Inport  Port=3
  Four_Rooms : Subsystem  VariantControl=CONTROLLER_ID ~= 4
  Single_Room : Subsystem  VariantControl=CONTROLLER_ID == 4
  T_room : Outport

== system MaIA_SDCI_Temperature_Control/Plant/Block_Based/Building Configuration/Four_Rooms ==
  Q_heat : Inport
  T_a : Inport  Port=2
  T_dist : Inport  Port=3
  Demux : Demux
  Demux1 : Demux
  Mux : Mux
  Mux1 : Mux
  Room 1 : Subsystem
  Room 2 : Subsystem
      settings: PortSchema="{\"entries\":[{\"content\":{\"sides\":[{\"content\":{\"connectorIds\":[\"In1\",\"In2\",\"In3\"]},\"type\":\"ConnectorPlacement.EquallySpacedRectSide\",\"uuid\":\"0a2b68a7-6c78-44f4-87c7-030cb71ece2c\"},{\"content\":{\"connectorIds\":[\"Out1\"],\"side\":\"RIGHT\"},\"type\":\"ConnectorPlacement.EquallySpacedRectSide\",\"uuid\":\"de932b4a-49c8-481c-bbfd-3e9145ee6205\"},{\"content\":{\"connectorIds\":[\"In4\"],\"side\":\"TOP\"},\"type\":\"ConnectorPlacement.EquallySpacedRectSide\",\"uuid\":\"d44a7c15-9f35-4c16-a0ff-1d853741c297\"}]},\"type\":\"ConnectorPlacement.EquallySpacedConnector\",\"uuid\":\"04a52546-fb89-43e8-987e-8ad3f7fcee3d\"}],\"packageUris\":[\"http://schema.mathworks.com/mf0/Connector/R2020b\"],\"version\":\"1.0\"}"
  Room 3 : Subsystem
      settings: PortSchema="{\"entries\":[{\"content\":{\"sides\":[{\"content\":{\"connectorIds\":[\"In1\",\"In2\",\"In3\"]},\"type\":\"ConnectorPlacement.EquallySpacedRectSide\",\"uuid\":\"0a2b68a7-6c78-44f4-87c7-030cb71ece2c\"},{\"content\":{\"connectorIds\":[\"Out1\"],\"side\":\"RIGHT\"},\"type\":\"ConnectorPlacement.EquallySpacedRectSide\",\"uuid\":\"de932b4a-49c8-481c-bbfd-3e9145ee6205\"},{\"content\":{\"connectorIds\":[\"In4\"],\"side\":\"TOP\"},\"type\":\"ConnectorPlacement.EquallySpacedRectSide\",\"uuid\":\"d44a7c15-9f35-4c16-a0ff-1d853741c297\"}]},\"type\":\"ConnectorPlacement.EquallySpacedConnector\",\"uuid\":\"04a52546-fb89-43e8-987e-8ad3f7fcee3d\"}],\"packageUris\":[\"http://schema.mathworks.com/mf0/Connector/R2020b\"],\"version\":\"1.0\"}"
  Room 4 : Subsystem
      settings: PortSchema="{\"entries\":[{\"content\":{\"sides\":[{\"content\":{\"connectorIds\":[\"In1\",\"In2\"]},\"type\":\"ConnectorPlacement.EquallySpacedRectSide\",\"uuid\":\"3123e626-39ae-4c5e-ad9d-71f2ee4166ba\"},{\"content\":{\"connectorIds\":[\"Out1\"],\"side\":\"RIGHT\"},\"type\":\"ConnectorPlacement.EquallySpacedRectSide\",\"uuid\":\"83543aab-31b5-42d7-bfd1-47f9acb0a83e\"},{\"content\":{\"connectorIds\":[\"In3\"],\"side\":\"TOP\"},\"type\":\"ConnectorPlacement.EquallySpacedRectSide\",\"uuid\":\"0f438efb-5d42-4db0-b0c2-140d5da12992\"}]},\"type\":\"ConnectorPlacement.EquallySpacedConnector\",\"uuid\":\"188efdfe-3b9a-4ae7-9956-cb99736032d7\"}],\"packageUris\":[\"http://schema.mathworks.com/mf0/Connector/R2020b\"],\"version\":\"1.0\"}"
  Sum : Sum  Inputs=|++
  T_room : Outport
  wires:
  Demux/1 -> Room 1/1(Q_1)  "Q_1"
  Demux/2 -> Room 2/1(Q_2)  "Q_2"
  Demux/3 -> Room 3/1(Q_3)  "Q_3"
  Demux/4 -> Room 4/1(Q_4)  "Q_4"
  T_a/1 -> Mux/4, Mux/3, Mux/1, Mux/2
  Mux/1 -> Sum/2  "T_a_nominal"
  T_dist/1 -> Sum/1
  Sum/1 -> Demux1/1  "T_a_effective"
  Demux1/1 -> Room 1/2(T_a_1)  "T_a_1"
  Demux1/2 -> Room 2/2(T_a_2)  "T_a_2"
  Demux1/3 -> Room 3/2(T_a_3)  "T_a_3"
  Demux1/4 -> Room 4/2(T_a_4)  "T_a_4"
  Q_heat/1 -> Demux/1
  Room 1/1(T_1) -> Room 2/4(T_1), Mux1/1
  Room 2/1(T_2) -> Room 1/3(T_2), Room 3/4(T_2), Mux1/2
  Room 3/1(T_3) -> Room 4/3(T_3), Mux1/3, Room 2/3(T_3)
  Room 4/1(T_4) -> Room 3/3(T_4), Mux1/4
  Mux1/1 -> T_room/1

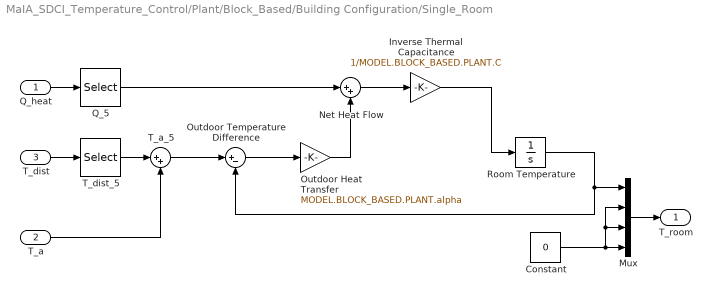
== system MaIA_SDCI_Temperature_Control/Plant/Block_Based/Building Configuration/Single_Room ==
  Q_heat : Inport
  T_a : Inport  Port=2
  T_dist : Inport  Port=3
  Constant : Constant  Value=0
  Inverse Thermal Capacitance : Gain  Gain=1/MODEL.BLOCK_BASED.PLANT.C
  Mux : Mux
  Net Heat Flow : Sum  Inputs=|++
  Outdoor Heat Transfer : Gain  Gain=MODEL.BLOCK_BASED.PLANT.alpha
  Outdoor Temperature Difference : Sum  Inputs=|+-
  Q_5 : Selector  InputPortWidth=4  IndexOptions=Index vector (dialog)  Indices=1  OutputSizes=1
  Room Temperature : Integrator  InitialCondition=MODEL.BLOCK_BASED.PLANT.initialTemperatureSingleRoom
  T_a_5 : Sum  Inputs=|++
  T_dist_5 : Selector  InputPortWidth=4  IndexOptions=Index vector (dialog)  Indices=1  OutputSizes=1
  T_room : Outport
  wires:
  Q_heat/1 -> Q_5/1
  T_dist/1 -> T_dist_5/1
  T_a/1 -> T_a_5/2
  T_dist_5/1 -> T_a_5/1
  T_a_5/1 -> Outdoor Temperature Difference/1
  Room Temperature/1 -> Outdoor Temperature Difference/2, Mux/1
  Outdoor Temperature Difference/1 -> Outdoor Heat Transfer/1
  Outdoor Heat Transfer/1 -> Net Heat Flow/2
  Q_5/1 -> Net Heat Flow/1
  Net Heat Flow/1 -> Inverse Thermal Capacitance/1
  Inverse Thermal Capacitance/1 -> Room Temperature/1
  Constant/1 -> Mux/2, Mux/3, Mux/4
  Mux/1 -> T_room/1

== system MaIA_SDCI_Temperature_Control/Plant/Physics_Based/Building Configuration/Four_Rooms ==
  Q_heat : Inport
  T_a : Inport  Port=2
  T_dist : Inport  Port=3
  Demux : Demux
  Demux1 : Demux
  Mux : Mux
  Mux1 : Mux
  Room 1 : Subsystem
  Room 2 : Subsystem
      settings: PortSchema="{\"entries\":[{\"content\":{\"sides\":[{\"content\":{\"connectorIds\":[\"In1\",\"In2\",\"In3\"]},\"type\":\"ConnectorPlacement.EquallySpacedRectSide\",\"uuid\":\"0a2b68a7-6c78-44f4-87c7-030cb71ece2c\"},{\"content\":{\"connectorIds\":[\"Out1\"],\"side\":\"RIGHT\"},\"type\":\"ConnectorPlacement.EquallySpacedRectSide\",\"uuid\":\"de932b4a-49c8-481c-bbfd-3e9145ee6205\"},{\"content\":{\"connectorIds\":[\"In4\"],\"side\":\"TOP\"},\"type\":\"ConnectorPlacement.EquallySpacedRectSide\",\"uuid\":\"d44a7c15-9f35-4c16-a0ff-1d853741c297\"}]},\"type\":\"ConnectorPlacement.EquallySpacedConnector\",\"uuid\":\"04a52546-fb89-43e8-987e-8ad3f7fcee3d\"}],\"packageUris\":[\"http://schema.mathworks.com/mf0/Connector/R2020b\"],\"version\":\"1.0\"}"
  Room 3 : Subsystem
      settings: PortSchema="{\"entries\":[{\"content\":{\"sides\":[{\"content\":{\"connectorIds\":[\"In1\",\"In2\",\"In3\"]},\"type\":\"ConnectorPlacement.EquallySpacedRectSide\",\"uuid\":\"0a2b68a7-6c78-44f4-87c7-030cb71ece2c\"},{\"content\":{\"connectorIds\":[\"Out1\"],\"side\":\"RIGHT\"},\"type\":\"ConnectorPlacement.EquallySpacedRectSide\",\"uuid\":\"de932b4a-49c8-481c-bbfd-3e9145ee6205\"},{\"content\":{\"connectorIds\":[\"In4\"],\"side\":\"TOP\"},\"type\":\"ConnectorPlacement.EquallySpacedRectSide\",\"uuid\":\"d44a7c15-9f35-4c16-a0ff-1d853741c297\"}]},\"type\":\"ConnectorPlacement.EquallySpacedConnector\",\"uuid\":\"04a52546-fb89-43e8-987e-8ad3f7fcee3d\"}],\"packageUris\":[\"http://schema.mathworks.com/mf0/Connector/R2020b\"],\"version\":\"1.0\"}"
  Room 4 : Subsystem
      settings: PortSchema="{\"entries\":[{\"content\":{\"sides\":[{\"content\":{\"connectorIds\":[\"In1\",\"In2\"]},\"type\":\"ConnectorPlacement.EquallySpacedRectSide\",\"uuid\":\"3123e626-39ae-4c5e-ad9d-71f2ee4166ba\"},{\"content\":{\"connectorIds\":[\"Out1\"],\"side\":\"RIGHT\"},\"type\":\"ConnectorPlacement.EquallySpacedRectSide\",\"uuid\":\"83543aab-31b5-42d7-bfd1-47f9acb0a83e\"},{\"content\":{\"connectorIds\":[\"In3\"],\"side\":\"TOP\"},\"type\":\"ConnectorPlacement.EquallySpacedRectSide\",\"uuid\":\"0f438efb-5d42-4db0-b0c2-140d5da12992\"}]},\"type\":\"ConnectorPlacement.EquallySpacedConnector\",\"uuid\":\"188efdfe-3b9a-4ae7-9956-cb99736032d7\"}],\"packageUris\":[\"http://schema.mathworks.com/mf0/Connector/R2020b\"],\"version\":\"1.0\"}"
  Sum : Sum  Inputs=|++
  T_room : Outport
  wires:
  Room 1/1(T_1) -> Mux1/1, Room 2/4(T_1)
  Demux1/3 -> Room 3/2(T_a_3)  "T_a_3"
  Room 4/1(T_4) -> Mux1/4, Room 3/3(T_4)
  Demux/4 -> Room 4/1(Q_4)  "Q_4"
  Room 2/1(T_2) -> Room 1/3(T_2), Mux1/2, Room 3/4(T_2)
  Demux1/1 -> Room 1/2(T_a_1)  "T_a_1"
  Demux1/2 -> Room 2/2(T_a_2)  "T_a_2"
  Demux/2 -> Room 2/1(Q_2)  "Q_2"
  Sum/1 -> Demux1/1  "T_a_effective"
  Room 3/1(T_3) -> Room 2/3(T_3), Mux1/3, Room 4/3(T_3)
  T_a/1 -> Mux/4, Mux/3, Mux/1, Mux/2
  Q_heat/1 -> Demux/1
  Mux1/1 -> T_room/1
  Demux1/4 -> Room 4/2(T_a_4)  "T_a_4"
  Mux/1 -> Sum/2  "T_a_nominal"
  Demux/3 -> Room 3/1(Q_3)  "Q_3"
  Demux/1 -> Room 1/1(Q_1)  "Q_1"
  T_dist/1 -> Sum/1

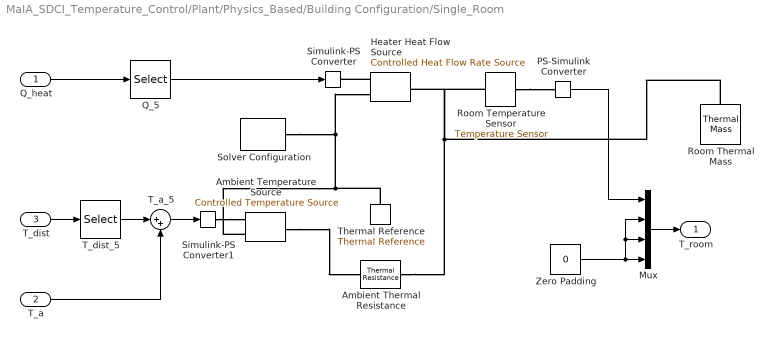
== system MaIA_SDCI_Temperature_Control/Plant/Physics_Based/Building Configuration/Single_Room ==
  Q_heat : Inport
  T_a : Inport  Port=2
  T_dist : Inport  Port=3
  " Thermal Reference" : fl_lib/Thermal/Thermal Elements/Thermal Reference
  Ambient Temperature Source : fl_lib/Thermal/Thermal Sources/Controlled Temperature Source
  Ambient Thermal Resistance : fl_lib/Thermal/Thermal Elements/Thermal Resistance  resistance=1/MODEL.SIMSCAPE.PLANT.alpha K/W  T_specify=off  T_priority=None  T=0 K  T_nominal_specify=off  T_nominal_value=1  T_nominal_unit=K  Q_specify=off  Q_priority=None  Q=0 W  Q_nominal_specify=off  Q_nominal_value=1  Q_nominal_unit=W
  "Heater Heat Flow Source " : fl_lib/Thermal/Thermal Sources/Controlled Heat Flow Rate Source
  Mux : Mux
  PS-Simulink Converter : nesl_utility/PS-Simulink Converter  PhysicalDomain=network_engine_domain  SubClassName=ps_output  LeftPortType=input  RightPortType=output  PseudoPeriodic=off  Frequencies=[]  VectorFormat=inherit  Unit=degC  AffineConversion=on
  Q_5 : Selector  InputPortWidth=4  IndexOptions=Index vector (dialog)  Indices=1  OutputSizes=1
  Room Temperature Sensor : fl_lib/Thermal/Thermal Sensors/Temperature Sensor  temperature_measure=foundation.enum.MeasurementReference.absolute
      settings: InternalSimscapePortConfiguration="{\"Bottom\":[],\"Left\":[{\"id\":\"A\",\"label\":\"A\",\"type\":\"foundation.thermal.thermal\"}],\"Right\":[{\"id\":\"T\",\"label\":\"T\",\"type\":\"output\"}],\"Top\":[]}"
  Room Thermal Mass : fl_lib/Thermal/Thermal Elements/Thermal Mass  mass_type=foundation.enum.constant_variable.constant  mass=1 kg  sp_heat=MODEL.SIMSCAPE.PLANT.C J/(K*kg)  mass_min=1e-6 kg  num_ports=foundation.enum.numPorts2.one  m_specify=off  m_priority=High  m=1 kg  m_nominal_specify=off  m_nominal_value=1  m_nominal_unit=kg  T_specify=on  T_priority=High  T=MODEL.SIMSCAPE.PLANT.initialTemperatureSingleRoom degC  T_nominal_specify=off  T_nominal_value=1  T_nominal_unit=K  Q_specify=off  Q_priority=None  Q=0 W  Q_nominal_specify=off  Q_nominal_value=1  Q_nominal_unit=W
  Simulink-PS Converter : nesl_utility/Simulink-PS Converter  PhysicalDomain=network_engine_domain  SubClassName=ps_input  LeftPortType=input  RightPortType=output  PseudoPeriodic=off  Frequencies=[]  NoiseDistribution=none  NoiseParameters=[]  Unit=W  AffineConversion=off  FilteringAndDerivatives=provide  SimscapeFilterOrder=1  InputFilterTimeConstant=0.001  UdotUserProvided=0
  Simulink-PS Converter1 : nesl_utility/Simulink-PS Converter  PhysicalDomain=network_engine_domain  SubClassName=ps_input  LeftPortType=input  RightPortType=output  PseudoPeriodic=off  Frequencies=[]  NoiseDistribution=none  NoiseParameters=[]  Unit=degC  AffineConversion=on  FilteringAndDerivatives=provide  SimscapeFilterOrder=1  InputFilterTimeConstant=0.001  UdotUserProvided=0
  "Solver Configuration " : nesl_utility/Solver Configuration  PhysicalDomain=network_engine_domain  SubClassName=solver  LeftPortType=input  RightPortType=generic  Tones=[]  Harmonics=[]  SimulateNoise=off  Profile=off  UseLocalSampling=off  EnableSwitchedLinearOptims=on  FrequencyDomain=off  UseCCode=off  RelTol=0.001  AbsTol=0.001  MinStep=1e-09  ToWorkspace=off  RevertToSquareIcSolve=off  NumHomotopyIterations=100  PhasorMode=off  PhasorModeNumHarmonics=1  ConsistencySolver=NEWTON_XTOL_AFTER_FTOL  IndexReductionMethod=DerivativeReplacement  DoDC=off  ResidualTolerance=1e-09  ConsistencyTolSource=GLOBAL  ConsistencyAbsTol=0.001  ConsistencyRelTol=0.001  ConsistencyTolFactor=0.001  UseLocalSolver=off  LocalSolverChoice=NE_BACKWARD_EULER_ADVANCER  ResolveIndetEquations=on  FunctionEvalNumThread=1  LocalSolverSampleTime=0.001  DoFixedCost=off  MaxNonlinIter=3  MaxModeIter=2  ComputeImpulses=off  ImpulseIterations=2  LinearAlgebra=auto  LinearAlgebraNumThread=0  EquationFormulation=NE_TIME_EF  DelaysMemoryBudget=1024  AutomaticFiltering=on  FilteringTimeConstant=0.001  PartitionStorageMethod=AS_NEEDED  PartitionMemoryBudget=1024  PartitionMethod=ROBUST  MultibodyUseLocalSolver=off  MultibodyLocalSolverChoice=ODE1  MultibodyLocalSolverSampleTime=0.001
  T_a_5 : Sum  Inputs=|++
  T_dist_5 : Selector  InputPortWidth=4  IndexOptions=Index vector (dialog)  Indices=1  OutputSizes=1
  Zero Padding : Constant  Value=0
  T_room : Outport
  wires:
  T_a/1 -> T_a_5/2
  Mux/1 -> T_room/1
  Q_heat/1 -> Q_5/1
  T_dist/1 -> T_dist_5/1
  T_dist_5/1 -> T_a_5/1
  Zero Padding/1 -> Mux/2, Mux/3, Mux/4
  Q_5/1 -> Simulink-PS Converter/1
  T_a_5/1 -> Simulink-PS Converter1/1
  PS-Simulink Converter/1 -> Mux/1
  connections:
  Ambient Temperature Source/RConn2 -- " Thermal Reference"/LConn1 -- "Solver Configuration "/RConn1 -- "Heater Heat Flow Source "/RConn2
  Ambient Thermal Resistance/RConn1 -- Room Thermal Mass/LConn1 -- Room Temperature Sensor/LConn1 -- "Heater Heat Flow Source "/LConn1
  Simulink-PS Converter1/RConn1 -- Ambient Temperature Source/RConn1
  Ambient Temperature Source/LConn1 -- Ambient Thermal Resistance/LConn1
  "Heater Heat Flow Source "/RConn1 -- Simulink-PS Converter/RConn1
  Room Temperature Sensor/RConn1 -- PS-Simulink Converter/LConn1

== system MaIA_SDCI_Temperature_Control/Plant/Block_Based/Building Configuration/Four_Rooms/Room 1 ==
  Q_1 : Inport
  T_a_1 : Inport  Port=2
  T_2 : Inport  Port=3
  Inverse Thermal Capacitance : Gain  Gain=1/MODEL.BLOCK_BASED.PLANT.C
  Neighbor 2 Heat Transfer : Gain  Gain=MODEL.BLOCK_BASED.PLANT.alpha
  Neighbor 2 Temperature Difference : Sum  Inputs=|+-
  Net Heat Flow : Sum  Inputs=|+++
  Outdoor Heat Transfer : Gain  Gain=MODEL.BLOCK_BASED.PLANT.alpha
  Outdoor Temperature Difference : Sum  Inputs=|+-
  Room Temperature : Integrator  InitialCondition=MODEL.BLOCK_BASED.PLANT.initialTemperature(1)
  T_1 : Outport
  wires:
  T_a_1/1 -> Outdoor Temperature Difference/1
  Room Temperature/1 -> Neighbor 2 Temperature Difference/2, T_1/1, Outdoor Temperature Difference/2
  Outdoor Temperature Difference/1 -> Outdoor Heat Transfer/1
  T_2/1 -> Neighbor 2 Temperature Difference/1
  Neighbor 2 Temperature Difference/1 -> Neighbor 2 Heat Transfer/1
  Outdoor Heat Transfer/1 -> Net Heat Flow/2
  Neighbor 2 Heat Transfer/1 -> Net Heat Flow/3
  Q_1/1 -> Net Heat Flow/1
  Net Heat Flow/1 -> Inverse Thermal Capacitance/1
  Inverse Thermal Capacitance/1 -> Room Temperature/1
